simulink model "TestMotorRotation"  (R2022a)
settings: Solver=VariableStepAuto  StartTime=0.0  StopTime=10.0  RelTol=1e-3
undefined symbols (not defined in the file): InputPWM, ticksPerRot, wheelR, WheelSpeed
libraries: arduinolib x8, spsEdgeDetectorLib x2, mobileRoboticsTrainingLib x1
settings Model: Creator=ryanj  LastModifiedBy=ryanj

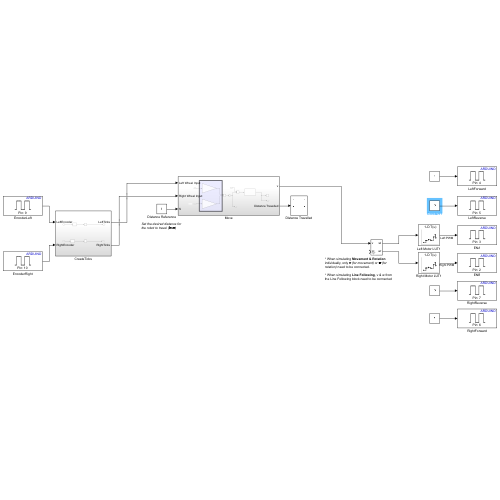
[thumbnail: Simulink's stored preview of the top-level diagram]
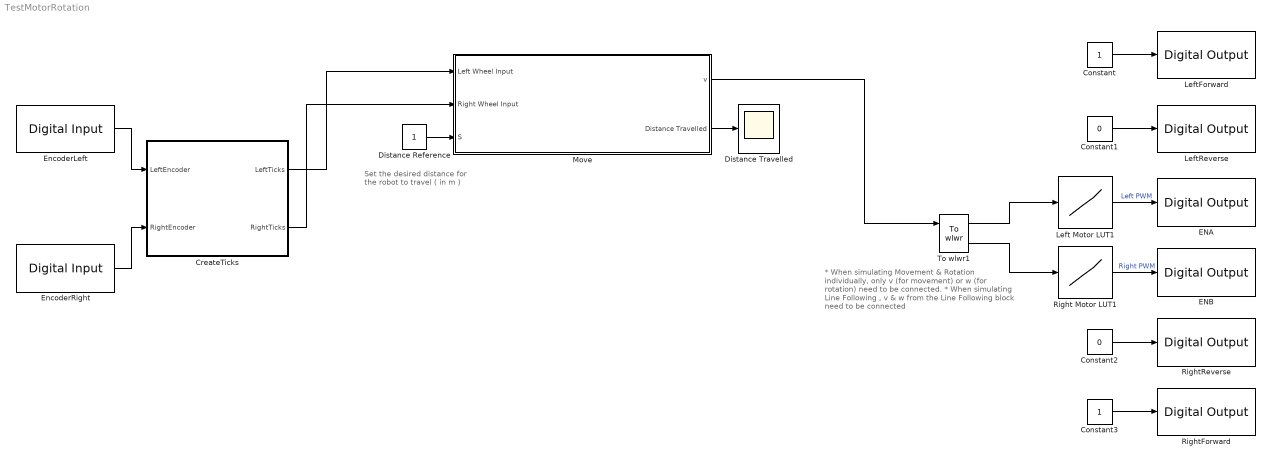
== system TestMotorRotation ==
  note: * When simulating Movement & Rotation individually, only v (for movement) or w (for rotation) need to be connected.
      |
      | * When simulating Line Following , v & w from the Line Following block need to be connected
  note: Set the desired distance for
      | the robot to travel ( in m )
  Constant : Constant
  Constant1 : Constant  Value=0
  Constant2 : Constant  Value=0
  Constant3 : Constant
  CreateTicks : Subsystem
  Distance Reference : Constant
  Distance Travelled : Scope
  ENA : arduinolib/Digital Output  pinNumber=3  Direction=output  blockPlatform=arduino
  ENB : arduinolib/Digital Output  pinNumber=2  Direction=output  blockPlatform=arduino
  EncoderLeft : arduinolib/Digital Input  pinNumber=9  mode=Default  Direction=input  SampleTime=0.1  blockPlatform=arduino
  EncoderRight : arduinolib/Digital Input  pinNumber=10  mode=Default  Direction=input  SampleTime=0.1  blockPlatform=arduino
  Left Motor LUT1 : Lookup_n-D  NumberOfTableDimensions=1  BreakpointsForDimension1=WheelSpeed  Table=InputPWM  InterpMethod=Nearest  ExtrapMethod=Clip  InternalRulePriority=Speed  RndMeth=Simplest
  LeftForward : arduinolib/Digital Output  pinNumber=4  Direction=output  blockPlatform=arduino
  LeftReverse : arduinolib/Digital Output  pinNumber=5  Direction=output  blockPlatform=arduino
  Move : Subsystem
  Right Motor LUT1 : Lookup_n-D  NumberOfTableDimensions=1  BreakpointsForDimension1=WheelSpeed  Table=InputPWM  InterpMethod=Nearest  ExtrapMethod=Clip  InternalRulePriority=Speed  RndMeth=Simplest
  RightForward : arduinolib/Digital Output  pinNumber=6  Direction=output  blockPlatform=arduino
  RightReverse : arduinolib/Digital Output  pinNumber=7  Direction=output  blockPlatform=arduino
  To wlwr1 : mobileRoboticsTrainingLib/To wlwr  axleLength=0.1  wheelR=0.05
  wires:
  Move/2(Distance Travelled) -> Distance Travelled/1
  CreateTicks/2(RightTicks) -> Move/2(Right Wheel Input)
  CreateTicks/1(LeftTicks) -> Move/1(Left Wheel Input)
  EncoderRight/1 -> CreateTicks/2(RightEncoder)
  EncoderLeft/1 -> CreateTicks/1(LeftEncoder)
  Left Motor LUT1/1 -> ENA/1  "Left PWM"
  To wlwr1/1 -> Left Motor LUT1/1
  To wlwr1/2 -> Right Motor LUT1/1
  Right Motor LUT1/1 -> ENB/1  "Right PWM"
  Distance Reference/1 -> Move/3(S)
  Move/1(v) -> To wlwr1/1
  Constant1/1 -> LeftReverse/1
  Constant/1 -> LeftForward/1
  Constant2/1 -> RightReverse/1
  Constant3/1 -> RightForward/1

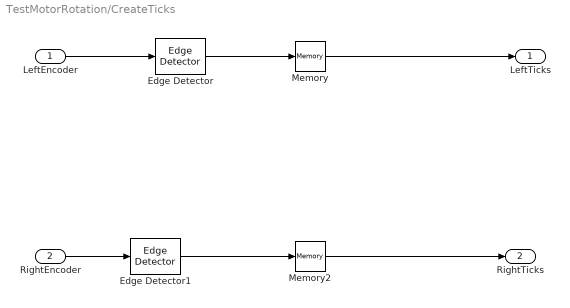
== system TestMotorRotation/CreateTicks ==
  LeftEncoder : Inport
  RightEncoder : Inport  Port=2
  Edge Detector : spsEdgeDetectorLib/Edge Detector  model=Rising  ic=0  Ts=0
      settings: SourceProductBaseCode=PS
  Edge Detector1 : spsEdgeDetectorLib/Edge Detector  model=Rising  ic=0  Ts=0
      settings: SourceProductBaseCode=PS
  Memory : Memory
  Memory2 : Memory
  LeftTicks : Outport
  RightTicks : Outport  Port=2
  wires:
  Memory/1 -> LeftTicks/1
  RightEncoder/1 -> Edge Detector1/1
  LeftEncoder/1 -> Edge Detector/1
  Edge Detector/1 -> Memory/1
  Edge Detector1/1 -> Memory2/1
  Memory2/1 -> RightTicks/1

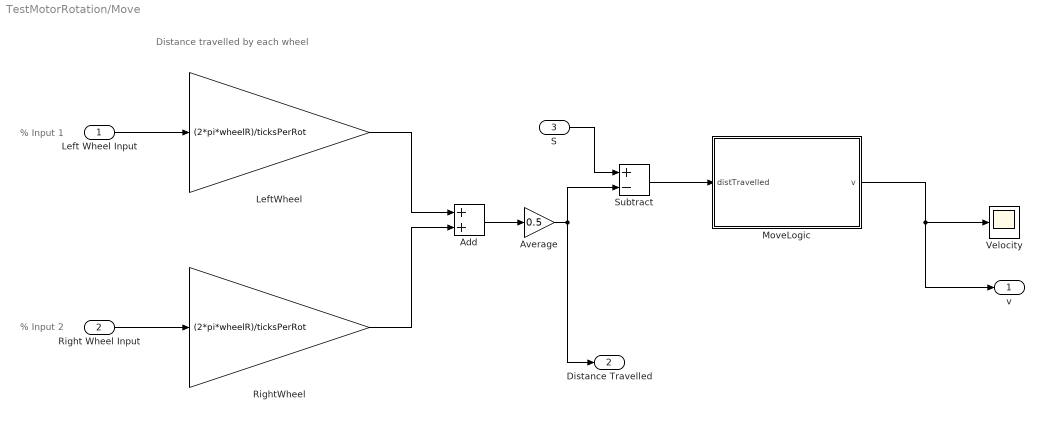
== system TestMotorRotation/Move ==
  note: Distance travelled by each wheel
  note: % Input 1
  note: % Input 2
  Left Wheel Input : Inport
  Right Wheel Input : Inport  Port=2
  S : Inport  Port=3
  Add : Sum
  Average : Gain  Gain=0.5
  LeftWheel : Gain  Gain=(2*pi*wheelR)/ticksPerRot
  MoveLogic : Stateflow chart  TreatAsAtomicUnit=on
  RightWheel : Gain  Gain=(2*pi*wheelR)/ticksPerRot
  Subtract : Sum  Inputs=+-
  Velocity : Scope
  v : Outport
  Distance Travelled : Outport  Port=2
  wires:
  Left Wheel Input/1 -> LeftWheel/1
  LeftWheel/1 -> Add/1
  Right Wheel Input/1 -> RightWheel/1
  S/1 -> Subtract/1
  RightWheel/1 -> Add/2
  Add/1 -> Average/1
  Average/1 -> Distance Travelled/1, Subtract/2
  Subtract/1 -> MoveLogic/1(distTravelled)
  MoveLogic/1(v) -> v/1, Velocity/1

== stateflow chart TestMotorRotation/Move/MoveLogic ==
  state MoveForward
    entry:
    v=0.1;
  state Stop
    entry:
    v=0;
  (default) -> MoveForward
  MoveForward -> Stop : [distTravelled <= 1]
  data: distTravelled input; v output
